simulink library "xpclib"  (Simulink 6.0)
settings: Solver=ode45  SolverMode=SingleTasking  StartTime=0.0  StopTime=10.0  RelTol=1e-3
values from neighbouring files (symbols this model uses):
  base = get_param( gcb, 'base' )    [maddiamondmm.m]    (also in maddiamondmm32frame.m; maddsmm16at.m; mdadsmm16at.m; mdiortddm64x0.m = hex2dec(addr(3:end)))
  block = find_system(bdroot,                          'FollowLinks', 'on',                          'LookUnderMasks', 'all',                          'MaskType', type )    [mdionipci6527.m]
  count = count + 1    (= 5)    [mdecodestate.m]
  port = get_param( gcb, 'port' )    [mdionipci6527.m]    (also in mdiortddm64x0.m = get_param(blocks{i}, 'port'))
undefined symbols (not defined in the file or in its folder): CIO, devid, DIO24, genixlib, get, handlers, irq, mbaseserialmask, mbwaudpmc, mdacbpcidas, mdiamondemeraldmask, mgenix, mmodemcontrol, mquamask, mrs232, msc150checks, mtargetboxleds, mtargetboxwatchdog, mxpccan, PCI, sizeof, vendid
libraries: xpclib x384, simulink x6
(part 6 of 7)

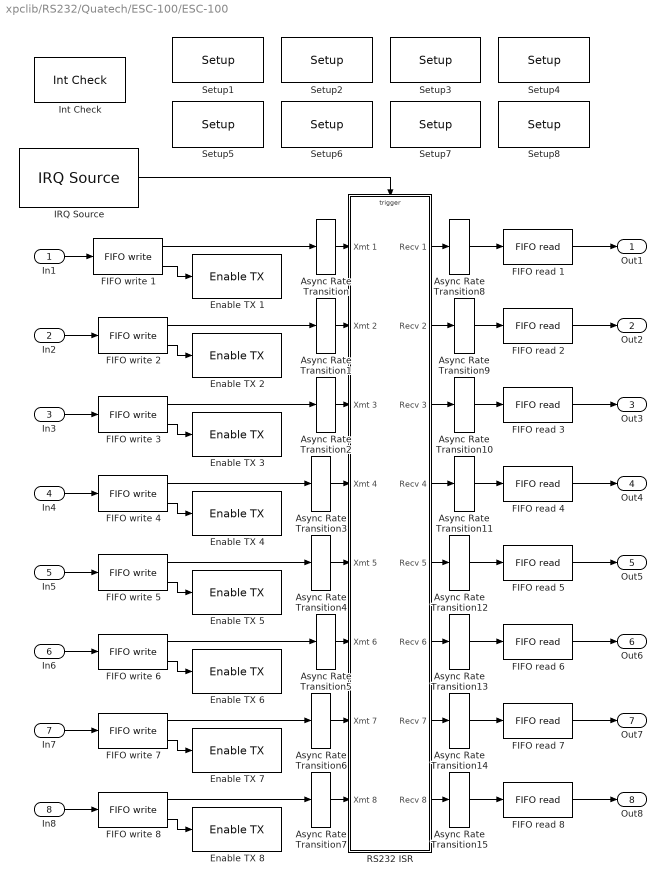
== system xpclib/RS232/Quatech/ESC-100/ESC-100 ==
  In1 : Inport  LatchInput=off
  In2 : Inport  Port=2  LatchInput=off
  In3 : Inport  Port=3  LatchInput=off
  In4 : Inport  Port=4  LatchInput=off
  In5 : Inport  Port=5  LatchInput=off
  In6 : Inport  Port=6  LatchInput=off
  In7 : Inport  Port=7  LatchInput=off
  In8 : Inport  Port=8  LatchInput=off
  Async Rate Transition{,1..15} (16 alike) : xpclib/Asynchronous Event/Async Rate Transition  sample_time=-1
  Enable TX 1 : xpclib/RS232/Quatech/ESC-100/ESC-100 Internal blocks/Enable TX   port=1  slot=brdslot
  Enable TX 2 : xpclib/RS232/Quatech/ESC-100/ESC-100 Internal blocks/Enable TX   port=2  slot=brdslot
  Enable TX 3 : xpclib/RS232/Quatech/ESC-100/ESC-100 Internal blocks/Enable TX   port=3  slot=brdslot
  Enable TX 4 : xpclib/RS232/Quatech/ESC-100/ESC-100 Internal blocks/Enable TX   port=4  slot=brdslot
  Enable TX 5 : xpclib/RS232/Quatech/ESC-100/ESC-100 Internal blocks/Enable TX   port=5  slot=brdslot
  Enable TX 6 : xpclib/RS232/Quatech/ESC-100/ESC-100 Internal blocks/Enable TX   port=6  slot=brdslot
  Enable TX 7 : xpclib/RS232/Quatech/ESC-100/ESC-100 Internal blocks/Enable TX   port=7  slot=brdslot
  Enable TX 8 : xpclib/RS232/Quatech/ESC-100/ESC-100 Internal blocks/Enable TX   port=8  slot=brdslot
  FIFO read {1..8} (8 alike) : xpclib/RS232/FIFO read   maxsize=1024  minsize=1  usedelimiter=on  delimiter=13  outputtype=count+16 bit uint  enable=off  enableout=off  sampletime=-1
  FIFO write 1 : xpclib/RS232/FIFO write   size=1024  inputtype=8 bit uint null terminated  present=on  sampletime=-1  id=XMT channel 1, IRQ 7
  FIFO write 2 : xpclib/RS232/FIFO write   size=1024  inputtype=8 bit uint null terminated  present=on  sampletime=-1  id=XMT channel 2, IRQ 7
  FIFO write 3 : xpclib/RS232/FIFO write   size=1024  inputtype=8 bit uint null terminated  present=on  sampletime=-1  id=XMT channel 3, IRQ 7
  FIFO write 4 : xpclib/RS232/FIFO write   size=1024  inputtype=8 bit uint null terminated  present=on  sampletime=-1  id=XMT channel 4, IRQ 7
  FIFO write 5 : xpclib/RS232/FIFO write   size=1024  inputtype=8 bit uint null terminated  present=on  sampletime=-1  id=XMT channel 5, IRQ 7
  FIFO write 6 : xpclib/RS232/FIFO write   size=1024  inputtype=8 bit uint null terminated  present=on  sampletime=-1  id=XMT channel 6, IRQ 7
  FIFO write 7 : xpclib/RS232/FIFO write   size=1024  inputtype=8 bit uint null terminated  present=on  sampletime=-1  id=XMT channel 7, IRQ 7
  FIFO write 8 : xpclib/RS232/FIFO write   size=1024  inputtype=8 bit uint null terminated  present=on  sampletime=-1  id=XMT channel 8, IRQ 7
  IRQ Source : xpclib/Asynchronous Event/IRQ Source  irqNo=7  preempt=off  b_type=None/Other  slot=brdslot
  Int Check : xpclib/RS232/Quatech/ESC-100/ESC-100 Internal blocks/Int Check  slot=brdslot  irqnum=7
  RS232 ISR : Subsystem  TreatAsAtomicUnit=on  PropExecContextAcrossSSBoundary=on  mask(RS232 ISR){slot=brdslot}
      mask help:
      | ESC-100
      | Quatech
      | Interrupt Service Routine
      mask init:
      | subslot = slot;
      mask Display:
      | disp('ESC-100\nISR');
      | port_label('input', 1, 'XMT1');
      | port_label('input', 2, 'XMT2');
      | port_label('input', 3, 'XMT3');
      | port_label('input', 4, 'XMT4');
      | port_label('input', 5, 'XMT5');
      | port_label('input', 6, 'XMT6');
      | port_label('input', 7, 'XMT7');
      | port_label('input', 8, 'XMT8');
      | port_label('output', 1, 'RCV1');
      | port_label('output', 2, 'RCV2');
      | port_label('output', 3, 'RCV3');
      | port_label('output', 4, 'RCV4');
      | port_label('output', 5, 'RCV5');
      | port_label('output', 6, 'RCV6');
      | port_label('output', 7, 'RCV7');
      | port_label('output', 8, 'RCV8');
  Setup1 : xpclib/RS232/Quatech/ESC-100/ESC-100 Internal blocks/Setup  port=1  baud=19200  width=8  nstop=1  parity=None  fmode=64 deep  rlevel=half full  ctsmode=on  slot=brdslot
  Setup2 : xpclib/RS232/Quatech/ESC-100/ESC-100 Internal blocks/Setup  port=2  baud=19200  width=8  nstop=1  parity=None  fmode=64 deep  rlevel=half full  ctsmode=on  slot=brdslot
  Setup3 : xpclib/RS232/Quatech/ESC-100/ESC-100 Internal blocks/Setup  port=3  baud=19200  width=8  nstop=1  parity=None  fmode=64 deep  rlevel=half full  ctsmode=on  slot=brdslot
  Setup4 : xpclib/RS232/Quatech/ESC-100/ESC-100 Internal blocks/Setup  port=4  baud=19200  width=8  nstop=1  parity=None  fmode=64 deep  rlevel=half full  ctsmode=on  slot=brdslot
  Setup5 : xpclib/RS232/Quatech/ESC-100/ESC-100 Internal blocks/Setup  port=5  baud=19200  width=8  nstop=1  parity=None  fmode=64 deep  rlevel=half full  ctsmode=on  slot=brdslot
  Setup6 : xpclib/RS232/Quatech/ESC-100/ESC-100 Internal blocks/Setup  port=6  baud=19200  width=8  nstop=1  parity=None  fmode=64 deep  rlevel=half full  ctsmode=on  slot=brdslot
  Setup7 : xpclib/RS232/Quatech/ESC-100/ESC-100 Internal blocks/Setup  port=7  baud=19200  width=8  nstop=1  parity=None  fmode=64 deep  rlevel=half full  ctsmode=on  slot=brdslot
  Setup8 : xpclib/RS232/Quatech/ESC-100/ESC-100 Internal blocks/Setup  port=8  baud=19200  width=8  nstop=1  parity=None  fmode=64 deep  rlevel=half full  ctsmode=on  slot=brdslot
  Out1 : Outport
  Out2 : Outport  Port=2
  Out3 : Outport  Port=3
  Out4 : Outport  Port=4
  Out5 : Outport  Port=5
  Out6 : Outport  Port=6
  Out7 : Outport  Port=7
  Out8 : Outport  Port=8
  wires:
  RS232 ISR/8(Recv 8) -> Async Rate Transition15/1
  RS232 ISR/7(Recv 7) -> Async Rate Transition14/1
  RS232 ISR/6(Recv 6) -> Async Rate Transition13/1
  RS232 ISR/5(Recv 5) -> Async Rate Transition12/1
  Async Rate Transition15/1 -> FIFO read 8/1
  FIFO read 8/1 -> Out8/1
  Async Rate Transition14/1 -> FIFO read 7/1
  FIFO read 7/1 -> Out7/1
  Async Rate Transition13/1 -> FIFO read 6/1
  FIFO read 6/1 -> Out6/1
  Async Rate Transition12/1 -> FIFO read 5/1
  FIFO read 5/1 -> Out5/1
  Async Rate Transition4/1 -> RS232 ISR/5(Xmt 5)
  Async Rate Transition5/1 -> RS232 ISR/6(Xmt 6)
  Async Rate Transition6/1 -> RS232 ISR/7(Xmt 7)
  Async Rate Transition7/1 -> RS232 ISR/8(Xmt 8)
  RS232 ISR/4(Recv 4) -> Async Rate Transition11/1
  Async Rate Transition1/1 -> RS232 ISR/2(Xmt 2)
  Async Rate Transition11/1 -> FIFO read 4/1
  Async Rate Transition10/1 -> FIFO read 3/1
  FIFO read 4/1 -> Out4/1
  FIFO read 3/1 -> Out3/1
  FIFO read 2/1 -> Out2/1
  Async Rate Transition9/1 -> FIFO read 2/1
  FIFO read 1/1 -> Out1/1
  Async Rate Transition8/1 -> FIFO read 1/1
  RS232 ISR/3(Recv 3) -> Async Rate Transition10/1
  RS232 ISR/2(Recv 2) -> Async Rate Transition9/1
  RS232 ISR/1(Recv 1) -> Async Rate Transition8/1
  Async Rate Transition3/1 -> RS232 ISR/4(Xmt 4)
  Async Rate Transition2/1 -> RS232 ISR/3(Xmt 3)
  Async Rate Transition/1 -> RS232 ISR/1(Xmt 1)
  IRQ Source/1 -> RS232 ISR/Trigger
  In1/1 -> FIFO write 1/1
  FIFO write 1/1 -> Async Rate Transition/1
  FIFO write 1/2 -> Enable TX 1/1
  FIFO write 2/1 -> Async Rate Transition1/1
  FIFO write 3/1 -> Async Rate Transition2/1
  FIFO write 4/1 -> Async Rate Transition3/1
  FIFO write 5/1 -> Async Rate Transition4/1
  FIFO write 6/1 -> Async Rate Transition5/1
  FIFO write 7/1 -> Async Rate Transition6/1
  FIFO write 8/1 -> Async Rate Transition7/1
  FIFO write 2/2 -> Enable TX 2/1
  FIFO write 3/2 -> Enable TX 3/1
  FIFO write 4/2 -> Enable TX 4/1
  FIFO write 5/2 -> Enable TX 5/1
  FIFO write 6/2 -> Enable TX 6/1
  FIFO write 7/2 -> Enable TX 7/1
  FIFO write 8/2 -> Enable TX 8/1
  In2/1 -> FIFO write 2/1
  In3/1 -> FIFO write 3/1
  In4/1 -> FIFO write 4/1
  In5/1 -> FIFO write 5/1
  In6/1 -> FIFO write 6/1
  In7/1 -> FIFO write 7/1
  In8/1 -> FIFO write 8/1

== system xpclib/RS232/Quatech/ESC-100/ESC-100 Internal blocks ==
  "Enable TX " : S-Function  FunctionName=sertxenable  Parameters=slot, port, 2  mask(Enable TX Int){port=1, slot=-1}
      mask prompts: slot "PCI slot: (-1 for autosearch)"
      mask help:
      | ESC-100
      | Quatech
      | Enable TX Interrupt
      mask Help: helpview(fullfile(docroot, 'mapfiles', 'xpc.map'), 'Quatech_Enable_Int')
      mask StyleString: popup(1|2|3|4|5|6|7|8),edit
      mask Display:
      | disp('ESC-100\nQuatech\nEnable TX int');
      | port_label('input', 1, 'E');
  Filter Int Reason : S-Function  FunctionName=filterqua  Parameters=port, 2, value  mask(Interrupt Source Filter){port=1, value=Transmitter empty}
      mask prompts: value "Filter value:"
      mask help:
      | ESC-100
      | Quatech
      | Interrupt Source Filter
      mask Help: helpview(fullfile(docroot, 'mapfiles', 'xpc.map'), 'Quatech_Filter_Ints')
      mask StyleString: popup(1|2|3|4|5|6|7|8),popup(Receive data|Transmitter empty|Modem status change)
      mask Display:
      | disp('ESC-100\nQuatech\nFilter Int Reason');
      | port_label('input', 1, 'S' );
      | port_label('output', 1, 'E' );
  Int Check : S-Function  FunctionName=intcheckqua  Parameters=slot, irqnum+4, boardtype,  mask(interrupt check){slot=-1, irqnum=5}
      mask prompts: slot "PCI slot: (-1 for autosearch)"; irqnum "IRQ Line Number"
      mask help:
      | ESC-100
      | Quatech
      | Interrupt Check
      mask init:
      | boardtype = 2;
      mask Help: helpview(fullfile(docroot, 'mapfiles', 'xpc.map'), 'Quatech_Interrupt_Check')
      mask StyleString: edit,popup(5|6|7|8|9|10|11|12|13|14|15)
      mask Display: disp('ESC-100\nQuatech\nInterrupt Check');
  Read HW FIFO : S-Function  FunctionName=serreadqua  Parameters=slot, port, 2, flush  mask(Read Data Port){port=1, flush=on, slot=-1}
      mask prompts: flush "Flush HW FIFO on startup"; slot "PCI slot: (-1 for autosearch)"
      mask help:
      | ESC-100
      | Quatech
      | Read Data Port
      mask Help: helpview(fullfile(docroot, 'mapfiles', 'xpc.map'), 'Quatech_Read_HW')
      mask StyleString: popup(1|2|3|4|5|6|7|8),checkbox,edit
      mask Display:
      | disp('ESC-100\nQuatech\nRead HW FIFO');
      | port_label('input', 1, 'E');
      | port_label('output', 1, 'D');
  Read Int Status : S-Function  FunctionName=iqueryqua  Parameters=slot, 2  mask(Interrupt Query){slot=-1}
      mask prompts: slot "PCI slot: (-1 for autosearch)"
      mask help:
      | ESC-100
      | Quatech
      | Interrupt Query
      mask Help: helpview(fullfile(docroot, 'mapfiles', 'xpc.map'), 'Quatech_Interrupt_Query')
      mask Display:
      | disp('ESC-100\nQuatech\nRead Int Status');
      | port_label('output', 1, 'S' );
  Setup : S-Function  FunctionName=setupqua  Parameters=slot, boardtype, port, baud, width, nstop, parity, fmode, ctsmode, rlevel  mask(setup){port=1, baud=115200, width=8, nstop=1, parity=None, fmode=64 deep, rlevel=half full, ctsmode=off, slot=-1}
      mask prompts: baud "Baud rate:"; width "Number of data bits:"; nstop "Number of stop bits:"; fmode "Fifo mode:"; rlevel "Receive trigger level:"; ctsmode "Enable auto RTS/CTS"; slot "PCI slot: (-1 for autosearch)"
      mask help:
      | ESC-100
      | Quatech
      | Setup
      mask init:
      | boardtype = 2;
      mask Help: helpview(fullfile(docroot, 'mapfiles', 'xpc.map'), 'Quatech_Setup')
      mask StyleString: popup(1|2|3|4|5|6|7|8),popup(921600|460800|230400|115200|57600|38400|19200|9600|4800|2400|1200|600|300|110),popup(5|6|7|8),popup(1|2),popup(None|Even|Odd|Mark|Space),popup(64 deep|16 deep|1 deep),popup(1|quarter full|half full|almost full),checkbox,edit
      mask Display: disp('ESC-100\nQuatech\nSetup')
  Write HW FIFO : S-Function  FunctionName=serwritequa  Parameters=slot, port, 2, 0  mask(Write Data Port){port=1, slot=-1}
      mask prompts: slot "PCI slot: (-1 for autosearch)"
      mask help:
      | ESC-100
      | Quatech
      | Write Data Port
      mask Help: helpview(fullfile(docroot, 'mapfiles', 'xpc.map'), 'Quatech_Write_HW')
      mask StyleString: popup(1|2|3|4|5|6|7|8),edit
      mask Display:
      | disp('ESC-100\nQuatech\nWrite HW FIFO');
      | port_label('input', 1, 'D');
      | port_label('input', 2, 'E');

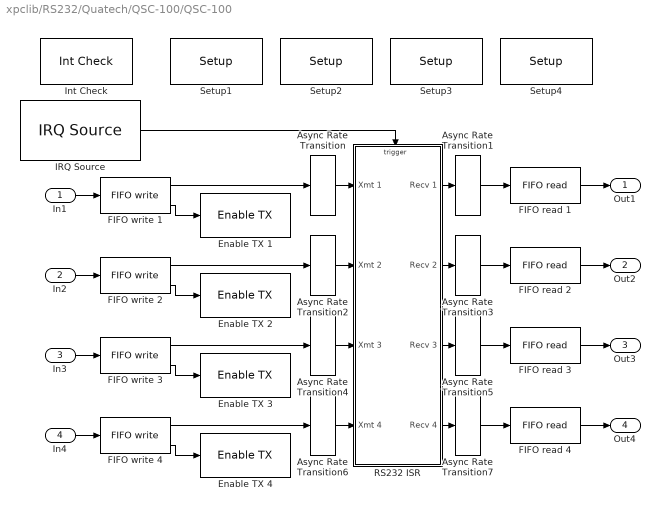
== system xpclib/RS232/Quatech/QSC-100/QSC-100 ==
  In1 : Inport  LatchInput=off
  In2 : Inport  Port=2  LatchInput=off
  In3 : Inport  Port=3  LatchInput=off
  In4 : Inport  Port=4  LatchInput=off
  Async Rate Transition{,1..7} (8 alike) : xpclib/Asynchronous Event/Async Rate Transition  sample_time=-1
  Enable TX 1 : xpclib/RS232/Quatech/QSC-100/QSC-100 Internal  blocks/Enable TX   port=1  slot=brdslot
  Enable TX 2 : xpclib/RS232/Quatech/QSC-100/QSC-100 Internal  blocks/Enable TX   port=2  slot=brdslot
  Enable TX 3 : xpclib/RS232/Quatech/QSC-100/QSC-100 Internal  blocks/Enable TX   port=3  slot=brdslot
  Enable TX 4 : xpclib/RS232/Quatech/QSC-100/QSC-100 Internal  blocks/Enable TX   port=4  slot=brdslot
  FIFO read {1..4} (4 alike) : xpclib/RS232/FIFO read   maxsize=1024  minsize=1  usedelimiter=on  delimiter=13  outputtype=count+16 bit uint  enable=off  enableout=off  sampletime=-1
  FIFO write 1 : xpclib/RS232/FIFO write   size=1024  inputtype=8 bit uint null terminated  present=on  sampletime=-1  id=XMT channel 1, IRQ 7
  FIFO write 2 : xpclib/RS232/FIFO write   size=1024  inputtype=8 bit uint null terminated  present=on  sampletime=-1  id=XMT channel 2, IRQ 7
  FIFO write 3 : xpclib/RS232/FIFO write   size=1024  inputtype=8 bit uint null terminated  present=on  sampletime=-1  id=XMT channel 3, IRQ 7
  FIFO write 4 : xpclib/RS232/FIFO write   size=1024  inputtype=8 bit uint null terminated  present=on  sampletime=-1  id=XMT channel 4, IRQ 7
  IRQ Source : xpclib/Asynchronous Event/IRQ Source  irqNo=7  preempt=off  b_type=None/Other  slot=brdslot
  Int Check : xpclib/RS232/Quatech/QSC-100/QSC-100 Internal  blocks/Int Check  slot=brdslot  irqnum=7
  RS232 ISR : Subsystem  TreatAsAtomicUnit=on  PropExecContextAcrossSSBoundary=on  mask(RS232 ISR){slot=brdslot}
      mask help:
      | QSC-100
      | Quatech
      | Interrupt Service Routine
      mask init:
      | subslot = slot;
      mask Display:
      | disp('QSC-100\nISR');
      | port_label('input', 1, 'XMT1');
      | port_label('input', 2, 'XMT2');
      | port_label('input', 3, 'XMT3');
      | port_label('input', 4, 'XMT4');
      | port_label('output', 1, 'RCV1');
      | port_label('output', 2, 'RCV2');
      | port_label('output', 3, 'RCV3');
      | port_label('output', 4, 'RCV4');
  Setup1 : xpclib/RS232/Quatech/QSC-100/QSC-100 Internal  blocks/Setup  port=1  baud=115200  width=8  nstop=1  parity=None  fmode=64 deep  rlevel=half full  ctsmode=on  slot=brdslot
  Setup2 : xpclib/RS232/Quatech/QSC-100/QSC-100 Internal  blocks/Setup  port=2  baud=115200  width=8  nstop=1  parity=None  fmode=64 deep  rlevel=half full  ctsmode=on  slot=brdslot
  Setup3 : xpclib/RS232/Quatech/QSC-100/QSC-100 Internal  blocks/Setup  port=3  baud=115200  width=8  nstop=1  parity=None  fmode=64 deep  rlevel=half full  ctsmode=on  slot=brdslot
  Setup4 : xpclib/RS232/Quatech/QSC-100/QSC-100 Internal  blocks/Setup  port=4  baud=115200  width=8  nstop=1  parity=None  fmode=64 deep  rlevel=half full  ctsmode=on  slot=brdslot
  Out1 : Outport
  Out2 : Outport  Port=2
  Out3 : Outport  Port=3
  Out4 : Outport  Port=4
  wires:
  FIFO write 1/2 -> Enable TX 1/1
  IRQ Source/1 -> RS232 ISR/Trigger
  Async Rate Transition/1 -> RS232 ISR/1(Xmt 1)
  Async Rate Transition4/1 -> RS232 ISR/3(Xmt 3)
  Async Rate Transition6/1 -> RS232 ISR/4(Xmt 4)
  RS232 ISR/1(Recv 1) -> Async Rate Transition1/1
  RS232 ISR/2(Recv 2) -> Async Rate Transition3/1
  RS232 ISR/3(Recv 3) -> Async Rate Transition5/1
  FIFO write 1/1 -> Async Rate Transition/1
  In1/1 -> FIFO write 1/1
  FIFO write 2/1 -> Async Rate Transition2/1
  FIFO write 3/1 -> Async Rate Transition4/1
  FIFO write 4/1 -> Async Rate Transition6/1
  In4/1 -> FIFO write 4/1
  In3/1 -> FIFO write 3/1
  In2/1 -> FIFO write 2/1
  Async Rate Transition1/1 -> FIFO read 1/1
  FIFO read 1/1 -> Out1/1
  Async Rate Transition3/1 -> FIFO read 2/1
  FIFO read 2/1 -> Out2/1
  FIFO read 3/1 -> Out3/1
  FIFO read 4/1 -> Out4/1
  Async Rate Transition5/1 -> FIFO read 3/1
  Async Rate Transition7/1 -> FIFO read 4/1
  FIFO write 2/2 -> Enable TX 2/1
  FIFO write 3/2 -> Enable TX 3/1
  FIFO write 4/2 -> Enable TX 4/1
  Async Rate Transition2/1 -> RS232 ISR/2(Xmt 2)
  RS232 ISR/4(Recv 4) -> Async Rate Transition7/1

== system xpclib/RS232/Quatech/QSC-100/QSC-100 Internal  blocks ==
  "Enable TX " : S-Function  FunctionName=sertxenable  Parameters=slot, port, 1  mask(Enable TX Int){port=1, slot=-1}
      mask prompts: slot "PCI slot: (-1 for autosearch)"
      mask help:
      | QSC-100
      | Quatech
      | Enable TX Interrupt
      mask Help: helpview(fullfile(docroot, 'mapfiles', 'xpc.map'), 'Quatech_Enable_Int')
      mask StyleString: popup(1|2|3|4),edit
      mask Display:
      | disp('QSC-100\nQuatech\nEnable TX int');
      | port_label('input', 1, 'E');
  Filter Int Reason : S-Function  FunctionName=filterqua  Parameters=port, 1, value  mask(Interrupt Source Filter){port=1, value=Receive data}
      mask prompts: value "Filter value:"
      mask help:
      | QSC-100
      | Quatech
      | Interrupt Source Filter
      mask Help: helpview(fullfile(docroot, 'mapfiles', 'xpc.map'), 'Quatech_Filter_Ints')
      mask StyleString: popup(1|2|3|4),popup(Receive data|Transmitter empty|Modem status change)
      mask Display:
      | disp('QSC-100\nQuatech\nFilter Int Reason');
      | port_label('input', 1, 'S' );
      | port_label('output', 1, 'E' );
  Int Check : S-Function  FunctionName=intcheckqua  Parameters=slot, irqnum+4, boardtype,  mask(interrupt check){slot=-1, irqnum=5}
      mask prompts: slot "PCI slot: (-1 for autosearch)"; irqnum "IRQ Line Number"
      mask help:
      | QSC-100
      | Quatech
      | Interrupt Check
      mask init:
      | boardtype = 1;
      mask Help: helpview(fullfile(docroot, 'mapfiles', 'xpc.map'), 'Quatech_Interrupt_Check')
      mask StyleString: edit,popup(5|6|7|8|9|10|11|12|13|14|15)
      mask Display: disp('QSC-100\nQuatech\nInterrupt Check');
  Read HW FIFO : S-Function  FunctionName=serreadqua  Parameters=slot, port, 1, flush  mask(Read Data Port){port=1, flush=on, slot=-1}
      mask prompts: flush "Flush HW FIFO on startup"; slot "PCI slot: (-1 for autosearch)"
      mask help:
      | QSC-100
      | Quatech
      | Read Data Port
      mask Help: helpview(fullfile(docroot, 'mapfiles', 'xpc.map'), 'Quatech_Read_HW')
      mask StyleString: popup(1|2|3|4),checkbox,edit
      mask Display:
      | disp('QSC-100\nQuatech\nRead HW FIFO');
      | port_label('input', 1, 'E');
      | port_label('output', 1, 'D');
  Read Int Status : S-Function  FunctionName=iqueryqua  Parameters=slot, 1  mask(Interrupt Query){slot=-1}
      mask prompts: slot "PCI slot: (-1 for autosearch)"
      mask help:
      | QSC-100
      | Quatech
      | Interrupt Query
      mask Help: helpview(fullfile(docroot, 'mapfiles', 'xpc.map'), 'Quatech_Interrupt_Query')
      mask Display:
      | disp('QSC-100\nQuatech\nRead Int Status');
      | port_label('output', 1, 'S' );
  Setup : S-Function  FunctionName=setupqua  Parameters=slot, boardtype, port, baud, width, nstop, parity, fmode, ctsmode, rlevel  mask(setup){port=1, baud=115200, width=8, nstop=1, parity=None, fmode=64 deep, rlevel=half full, ctsmode=off, slot=-1}
      mask prompts: baud "Baud rate:"; width "Number of data bits:"; nstop "Number of stop bits:"; fmode "Fifo mode:"; rlevel "Receive trigger level:"; ctsmode "Enable auto RTS/CTS"; slot "PCI slot: (-1 for autosearch)"
      mask help:
      | QSC-100
      | Quatech
      | Setup
      mask init:
      | boardtype = 1;
      mask Help: helpview(fullfile(docroot, 'mapfiles', 'xpc.map'), 'Quatech_Setup')
      mask StyleString: popup(1|2|3|4),popup(921600|460800|230400|115200|57600|38400|19200|9600|4800|2400|1200|600|300|110),popup(5|6|7|8),popup(1|2),popup(None|Even|Odd|Mark|Space),popup(64 deep|16 deep|1 deep),popup(1|quarter full|half full|almost full),checkbox,edit
      mask Display: disp('QSC-100\nQuatech\nSetup');
  Write HW FIFO : S-Function  FunctionName=serwritequa  Parameters=slot, port, 1, 0  mask(Write Data Port){port=1, slot=-1}
      mask prompts: slot "PCI slot: (-1 for autosearch)"
      mask help:
      | QSC-100
      | Quatech
      | Write Data Port
      mask Help: helpview(fullfile(docroot, 'mapfiles', 'xpc.map'), 'Quatech_Write_HW')
      mask StyleString: popup(1|2|3|4),edit
      mask Display:
      | disp('QSC-100\nQuatech\nWrite HW FIFO');
      | port_label('input', 1, 'D');
      | port_label('input', 2, 'E');

== system xpclib/RS232/Quatech/QSC-200/300/QSC-200/300 Internal  blocks1 ==
  "Enable TX " : S-Function  FunctionName=sertxenable  Parameters=slot, port, 3  mask(Enable TX Int){port=1, slot=-1}
      mask prompts: slot "PCI slot: (-1 for autosearch)"
      mask help:
      | QSC-200/300
      | Quatech
      | Enable TX Interrupt
      mask Help: helpview(fullfile(docroot, 'mapfiles', 'xpc.map'), 'Quatech_Enable_Int')
      mask StyleString: popup(1|2|3|4),edit
      mask Display:
      | disp('QSC-200/300\nQuatech\nEnable TX int');
      | port_label('input', 1, 'E');
  Filter Int Reason : S-Function  FunctionName=filterqua  Parameters=port, 3, value  mask(Interrupt Source Filter){port=1, value=Receive data}
      mask prompts: value "Filter value:"
      mask help:
      | QSC-200/300
      | Quatech
      | Interrupt Source Filter
      mask Help: helpview(fullfile(docroot, 'mapfiles', 'xpc.map'), 'Quatech_Filter_Ints')
      mask StyleString: popup(1|2|3|4),popup(Receive data|Transmitter empty|Modem status change)
      mask Display:
      | disp('QSC-200/300\nQuatech\nFilter Int Reason');
      | port_label('input', 1, 'S' );
      | port_label('output', 1, 'E' );
  Int Check : S-Function  FunctionName=intcheckqua  Parameters=slot, irqnum+4, boardtype,  mask(interrupt check){slot=-1, irqnum=5}
      mask prompts: slot "PCI slot: (-1 for autosearch)"; irqnum "IRQ Line Number"
      mask help:
      | QSC-200/300
      | Quatech
      | Interrupt Check
      mask init:
      | boardtype = 3;
      mask Help: helpview(fullfile(docroot, 'mapfiles', 'xpc.map'), 'Quatech_Interrupt_Check')
      mask StyleString: edit,popup(5|6|7|8|9|10|11|12|13|14|15)
      mask Display: disp('QSC-200/300\nQuatech\nInterrupt Check');
  Read HW FIFO : S-Function  FunctionName=serreadqua  Parameters=slot, port, 3, flush  mask(Read Data Port){port=1, flush=on, slot=-1}
      mask prompts: flush "Flush HW FIFO on startup"; slot "PCI slot: (-1 for autosearch)"
      mask help:
      | QSC-200/300
      | Quatech
      | Read Data Port
      mask Help: helpview(fullfile(docroot, 'mapfiles', 'xpc.map'), 'Quatech_Read_HW')
      mask StyleString: popup(1|2|3|4),checkbox,edit
      mask Display:
      | disp('QSC-200/300\nQuatech\nRead HW FIFO');
      | port_label('input', 1, 'E');
      | port_label('output', 1, 'D');
  Read Int Status : S-Function  FunctionName=iqueryqua  Parameters=slot, 3  mask(Interrupt Query){slot=-1}
      mask prompts: slot "PCI slot: (-1 for autosearch)"
      mask help:
      | QSC-200/300
      | Quatech
      | Interrupt Query
      mask Help: helpview(fullfile(docroot, 'mapfiles', 'xpc.map'), 'Quatech_Interrupt_Query')
      mask Display:
      | disp('QSC-200/300\nQuatech\nRead Int Status');
      | port_label('output', 1, 'S' );
  Setup : S-Function  FunctionName=setupqua  Parameters=slot, boardtype, port, baud, width, nstop, parity, fmode, ctsmode, rlevel  mask(setup){port=1, baud=115200, width=8, nstop=1, parity=None, fmode=64 deep, rlevel=half full, ctsmode=off, slot=-1}
      mask prompts: baud "Baud rate:"; width "Number of data bits:"; nstop "Number of stop bits:"; fmode "Fifo mode:"; rlevel "Receive trigger level:"; ctsmode "Enable auto RTS/CTS"; slot "PCI slot: (-1 for autosearch)"
      mask help:
      | QSC-200/300
      | Quatech
      | Setup
      mask init:
      | boardtype = 3;
      mask Help: helpview(fullfile(docroot, 'mapfiles', 'xpc.map'), 'Quatech_Setup')
      mask StyleString: popup(1|2|3|4),popup(921600|460800|230400|115200|57600|38400|19200|9600|4800|2400|1200|600|300|110),popup(5|6|7|8),popup(1|2),popup(None|Even|Odd|Mark|Space),popup(64 deep|16 deep|1 deep),popup(1|quarter full|half full|almost full),checkbox,edit
      mask Display: disp('QSC-200/300\nQuatech\nSetup');
  Write HW FIFO : S-Function  FunctionName=serwritequa  Parameters=slot, port, 3, onxmt  mask(Write Data Port){port=1, onxmt=None, slot=-1}
      mask prompts: onxmt "Assert on Transmit:"; slot "PCI slot: (-1 for autosearch)"
      mask help:
      | QSC-200/300
      | Quatech
      | Write Data Port
      mask Help: helpview(fullfile(docroot, 'mapfiles', 'xpc.map'), 'Quatech_Write_HW')
      mask StyleString: popup(1|2|3|4),popup(None|RTS|DTR),edit
      mask Display:
      | disp('QSC-200/300\nQuatech\nWrite HW FIFO');
      | port_label('input', 1, 'D');
      | port_label('input', 2, 'E');

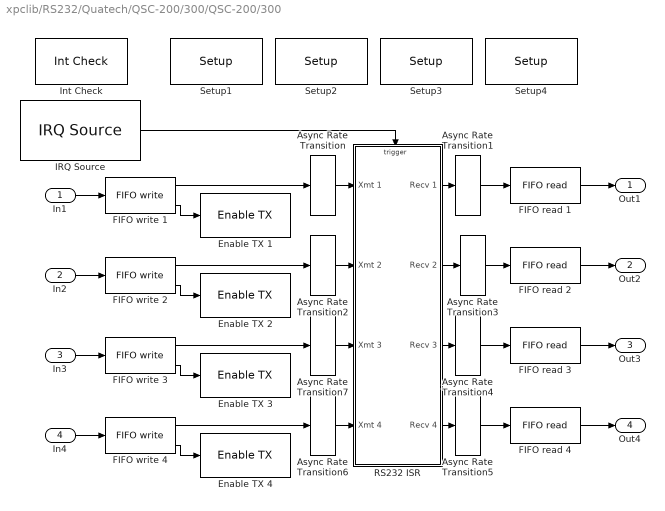
== system xpclib/RS232/Quatech/QSC-200/300/QSC-200/300  ==
  In1 : Inport  LatchInput=off
  In2 : Inport  Port=2  LatchInput=off
  In3 : Inport  Port=3  LatchInput=off
  In4 : Inport  Port=4  LatchInput=off
  Async Rate Transition{,1..7} (8 alike) : xpclib/Asynchronous Event/Async Rate Transition  sample_time=-1
  Enable TX 1 : xpclib/RS232/Quatech/QSC-200//300/QSC-200//300 Internal  blocks1/Enable TX   port=1  slot=brdslot
  Enable TX 2 : xpclib/RS232/Quatech/QSC-200//300/QSC-200//300 Internal  blocks1/Enable TX   port=2  slot=brdslot
  Enable TX 3 : xpclib/RS232/Quatech/QSC-200//300/QSC-200//300 Internal  blocks1/Enable TX   port=3  slot=brdslot
  Enable TX 4 : xpclib/RS232/Quatech/QSC-200//300/QSC-200//300 Internal  blocks1/Enable TX   port=4  slot=brdslot
  FIFO read {1..4} (4 alike) : xpclib/RS232/FIFO read   maxsize=1024  minsize=1  usedelimiter=on  delimiter=13  outputtype=count+16 bit uint  enable=off  enableout=off  sampletime=-1
  FIFO write {1..4} (4 alike) : xpclib/RS232/FIFO write   size=1024  inputtype=8 bit uint null terminated  present=on  sampletime=-1
  IRQ Source : xpclib/Asynchronous Event/IRQ Source  irqNo=7  preempt=off  b_type=None/Other  slot=brdslot
  Int Check : xpclib/RS232/Quatech/QSC-200//300/QSC-200//300 Internal  blocks1/Int Check  slot=brdslot  irqnum=7
  RS232 ISR : Subsystem  TreatAsAtomicUnit=on  PropExecContextAcrossSSBoundary=on  mask(RS232 ISR){slot=brdslot}
      mask help:
      | QSC-100
      | Quatech
      | Interrupt Service Routine
      mask init:
      | subslot = slot;
      mask Display:
      | disp('QSC-100\nISR');
      | port_label('input', 1, 'XMT1');
      | port_label('input', 2, 'XMT2');
      | port_label('input', 3, 'XMT3');
      | port_label('input', 4, 'XMT4');
      | port_label('output', 1, 'RCV1');
      | port_label('output', 2, 'RCV2');
      | port_label('output', 3, 'RCV3');
      | port_label('output', 4, 'RCV4');
  Setup1 : xpclib/RS232/Quatech/QSC-200//300/QSC-200//300 Internal  blocks1/Setup  port=1  baud=115200  width=8  nstop=1  parity=None  fmode=64 deep  rlevel=half full  ctsmode=on  slot=brdslot
  Setup2 : xpclib/RS232/Quatech/QSC-200//300/QSC-200//300 Internal  blocks1/Setup  port=2  baud=115200  width=8  nstop=1  parity=None  fmode=64 deep  rlevel=half full  ctsmode=on  slot=brdslot
  Setup3 : xpclib/RS232/Quatech/QSC-200//300/QSC-200//300 Internal  blocks1/Setup  port=3  baud=115200  width=8  nstop=1  parity=None  fmode=64 deep  rlevel=half full  ctsmode=on  slot=brdslot
  Setup4 : xpclib/RS232/Quatech/QSC-200//300/QSC-200//300 Internal  blocks1/Setup  port=4  baud=115200  width=8  nstop=1  parity=None  fmode=64 deep  rlevel=half full  ctsmode=on  slot=brdslot
  Out1 : Outport
  Out2 : Outport  Port=2
  Out3 : Outport  Port=3
  Out4 : Outport  Port=4
  wires:
  RS232 ISR/4(Recv 4) -> Async Rate Transition5/1
  Async Rate Transition2/1 -> RS232 ISR/2(Xmt 2)
  FIFO write 4/2 -> Enable TX 4/1
  FIFO write 3/2 -> Enable TX 3/1
  FIFO write 2/2 -> Enable TX 2/1
  FIFO read 4/1 -> Out4/1
  FIFO read 3/1 -> Out3/1
  FIFO read 2/1 -> Out2/1
  FIFO read 1/1 -> Out1/1
  Async Rate Transition1/1 -> FIFO read 1/1
  In2/1 -> FIFO write 2/1
  In3/1 -> FIFO write 3/1
  In4/1 -> FIFO write 4/1
  FIFO write 4/1 -> Async Rate Transition6/1
  FIFO write 3/1 -> Async Rate Transition7/1
  FIFO write 2/1 -> Async Rate Transition2/1
  In1/1 -> FIFO write 1/1
  FIFO write 1/1 -> Async Rate Transition/1
  RS232 ISR/3(Recv 3) -> Async Rate Transition4/1
  RS232 ISR/2(Recv 2) -> Async Rate Transition3/1
  RS232 ISR/1(Recv 1) -> Async Rate Transition1/1
  Async Rate Transition6/1 -> RS232 ISR/4(Xmt 4)
  Async Rate Transition7/1 -> RS232 ISR/3(Xmt 3)
  Async Rate Transition/1 -> RS232 ISR/1(Xmt 1)
  IRQ Source/1 -> RS232 ISR/Trigger
  FIFO write 1/2 -> Enable TX 1/1
  Async Rate Transition4/1 -> FIFO read 3/1
  Async Rate Transition5/1 -> FIFO read 4/1
  Async Rate Transition3/1 -> FIFO read 2/1

== system xpclib/RS232/Diamond/Emerald-MM /Diamond Emerald-MM Serial/RS232 ISR ==
  Xmt 1 : Inport  LatchInput=off
  Xmt 2 : Inport  Port=2  LatchInput=off
  Xmt 3 : Inport  Port=3  LatchInput=off
  Xmt 4 : Inport  Port=4  LatchInput=off
  function : TriggerPort  TriggerType=function-call
  While Iterator Subsystem : Subsystem  TreatAsAtomicUnit=on  PropExecContextAcrossSSBoundary=on
  Recv 1 : Outport
  Recv 2 : Outport  Port=2
  Recv 3 : Outport  Port=3
  Recv 4 : Outport  Port=4
  wires:
  While Iterator Subsystem/4(Recv 4) -> Recv 4/1
  While Iterator Subsystem/3(Recv 3) -> Recv 3/1
  Xmt 4/1 -> While Iterator Subsystem/4(Xmt 4)
  Xmt 3/1 -> While Iterator Subsystem/3(Xmt 3)
  While Iterator Subsystem/2(Recv 2) -> Recv 2/1
  While Iterator Subsystem/1(Recv 1) -> Recv 1/1
  Xmt 2/1 -> While Iterator Subsystem/2(Xmt 2)
  Xmt 1/1 -> While Iterator Subsystem/1(Xmt 1)

== system xpclib/RS232/Diamond/Emerald-MM8 /Diamond Emerald-MM8 Serial/RS232 ISR ==
  Xmt 1 : Inport  LatchInput=off
  Xmt 2 : Inport  Port=2  LatchInput=off
  Xmt 3 : Inport  Port=3  LatchInput=off
  Xmt 4 : Inport  Port=4  LatchInput=off
  Xmt 5 : Inport  Port=5  LatchInput=off
  Xmt 6 : Inport  Port=6  LatchInput=off
  Xmt 7 : Inport  Port=7  LatchInput=off
  Xmt 8 : Inport  Port=8  LatchInput=off
  function : TriggerPort  TriggerType=function-call
  While Iterator Subsystem : Subsystem  TreatAsAtomicUnit=on  PropExecContextAcrossSSBoundary=on
  Recv 1 : Outport
  Recv 2 : Outport  Port=2
  Recv 3 : Outport  Port=3
  Recv 4 : Outport  Port=4
  Recv 5 : Outport  Port=5
  Recv 6 : Outport  Port=6
  Recv 7 : Outport  Port=7
  Recv 8 : Outport  Port=8
  wires:
  Xmt 8/1 -> While Iterator Subsystem/8(Xmt 8)
  Xmt 7/1 -> While Iterator Subsystem/7(Xmt 7)
  Xmt 6/1 -> While Iterator Subsystem/6(Xmt 6)
  Xmt 5/1 -> While Iterator Subsystem/5(Xmt 5)
  While Iterator Subsystem/8(Recv 8) -> Recv 8/1
  While Iterator Subsystem/7(Recv 7) -> Recv 7/1
  While Iterator Subsystem/6(Recv 6) -> Recv 6/1
  While Iterator Subsystem/5(Recv 5) -> Recv 5/1
  While Iterator Subsystem/4(Recv 4) -> Recv 4/1
  While Iterator Subsystem/3(Recv 3) -> Recv 3/1
  Xmt 4/1 -> While Iterator Subsystem/4(Xmt 4)
  Xmt 3/1 -> While Iterator Subsystem/3(Xmt 3)
  While Iterator Subsystem/2(Recv 2) -> Recv 2/1
  While Iterator Subsystem/1(Recv 1) -> Recv 1/1
  Xmt 2/1 -> While Iterator Subsystem/2(Xmt 2)
  Xmt 1/1 -> While Iterator Subsystem/1(Xmt 1)

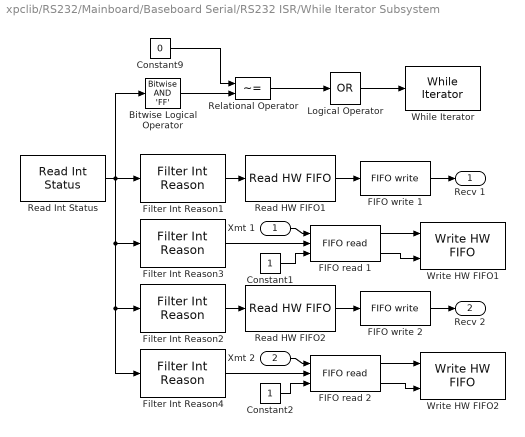
== system xpclib/RS232/Mainboard/Baseboard Serial/RS232 ISR/While Iterator Subsystem ==
  Xmt 1 : Inport  LatchInput=off
  Xmt 2 : Inport  Port=2  LatchInput=off
  Bitwise Logical Operator : simulink/Logic and Bit Operations/Bitwise Operator  logicop=AND  UseBitMask=on  BitMask='FF'  BitMaskRealWorld=Stored Integer
  Constant1 : Constant  OutDataTypeMode=uint32
  Constant2 : Constant  OutDataTypeMode=uint32
  Constant9 : Constant  Value=0  OutDataTypeMode=uint32
  FIFO read 1 : xpclib/RS232/FIFO read   maxsize=60  minsize=1  usedelimiter=off  delimiter=13  outputtype=count+32 bit uint  enable=on  enableout=on  sampletime=-1
  FIFO read 2 : xpclib/RS232/FIFO read   maxsize=60  minsize=1  usedelimiter=off  delimiter=13  outputtype=count+32 bit uint  enable=on  enableout=on  sampletime=-1
  FIFO write 1 : xpclib/RS232/FIFO write   size=1024  inputtype=count+32 bit uint  present=off  sampletime=-1  id=RCV channel 1, IRQ 4
  FIFO write 2 : xpclib/RS232/FIFO write   size=1024  inputtype=count+32 bit uint  present=off  sampletime=-1  id=RCV channel 2, IRQ 4
  Filter Int Reason1 : xpclib/RS232/Mainboard/Baseboard Serial Internal  blocks/Filter Int Reason  port=1  value=Receive data
  Filter Int Reason2 : xpclib/RS232/Mainboard/Baseboard Serial Internal  blocks/Filter Int Reason  port=2  value=Receive data
  Filter Int Reason3 : xpclib/RS232/Mainboard/Baseboard Serial Internal  blocks/Filter Int Reason  port=1  value=Transmitter empty
  Filter Int Reason4 : xpclib/RS232/Mainboard/Baseboard Serial Internal  blocks/Filter Int Reason  port=2  value=Transmitter empty
  Logical Operator : Logic  Operator=OR  Inputs=1  AllPortsSameDT=off
  Read HW FIFO1 : xpclib/RS232/Mainboard/Baseboard Serial Internal  blocks/Read HW FIFO  flush=on  addr=baddr1
  Read HW FIFO2 : xpclib/RS232/Mainboard/Baseboard Serial Internal  blocks/Read HW FIFO  flush=on  addr=baddr2
  Read Int Status : xpclib/RS232/Mainboard/Baseboard Serial Internal  blocks/Read Int Status  addr1=baddr1  addr2=baddr2
  Relational Operator : RelationalOperator  Operator=~=
  While Iterator : WhileIterator  MaxIters=65  WhileBlockType=do-while
  Write HW FIFO1 : xpclib/RS232/Mainboard/Baseboard Serial Internal  blocks/Write HW FIFO  addr=baddr1
  Write HW FIFO2 : xpclib/RS232/Mainboard/Baseboard Serial Internal  blocks/Write HW FIFO  addr=baddr2
  Recv 1 : Outport
  Recv 2 : Outport  Port=2
  wires:
  Read Int Status/1 -> Filter Int Reason1/1, Filter Int Reason3/1, Filter Int Reason4/1, Filter Int Reason2/1, Bitwise Logical Operator/1
  Filter Int Reason1/1 -> Read HW FIFO1/1
  FIFO write 1/1 -> Recv 1/1
  Read HW FIFO1/1 -> FIFO write 1/1
  Filter Int Reason3/1 -> FIFO read 1/2
  Xmt 1/1 -> FIFO read 1/1
  Filter Int Reason2/1 -> Read HW FIFO2/1
  FIFO write 2/1 -> Recv 2/1
  Read HW FIFO2/1 -> FIFO write 2/1
  Filter Int Reason4/1 -> FIFO read 2/2
  Xmt 2/1 -> FIFO read 2/1
  FIFO read 2/1 -> Write HW FIFO2/1
  FIFO read 2/2 -> Write HW FIFO2/2
  FIFO read 1/1 -> Write HW FIFO1/1
  FIFO read 1/2 -> Write HW FIFO1/2
  Constant1/1 -> FIFO read 1/3
  Constant2/1 -> FIFO read 2/3
  Logical Operator/1 -> While Iterator/1
  Relational Operator/1 -> Logical Operator/1
  Bitwise Logical Operator/1 -> Relational Operator/2
  Constant9/1 -> Relational Operator/1

== system xpclib/RS232/Quatech/ESC-100/ESC-100/RS232 ISR ==
  Xmt 1 : Inport  LatchInput=off
  Xmt 2 : Inport  Port=2  LatchInput=off
  Xmt 3 : Inport  Port=3  LatchInput=off
  Xmt 4 : Inport  Port=4  LatchInput=off
  Xmt 5 : Inport  Port=5  LatchInput=off
  Xmt 6 : Inport  Port=6  LatchInput=off
  Xmt 7 : Inport  Port=7  LatchInput=off
  Xmt 8 : Inport  Port=8  LatchInput=off
  function : TriggerPort  TriggerType=function-call
  While Iterator Subsystem : Subsystem  TreatAsAtomicUnit=on  PropExecContextAcrossSSBoundary=on
  Recv 1 : Outport
  Recv 2 : Outport  Port=2
  Recv 3 : Outport  Port=3
  Recv 4 : Outport  Port=4
  Recv 5 : Outport  Port=5
  Recv 6 : Outport  Port=6
  Recv 7 : Outport  Port=7
  Recv 8 : Outport  Port=8
  wires:
  Xmt 1/1 -> While Iterator Subsystem/1(Xmt 1)
  Xmt 2/1 -> While Iterator Subsystem/2(Xmt 2)
  Xmt 3/1 -> While Iterator Subsystem/3(Xmt 3)
  Xmt 4/1 -> While Iterator Subsystem/4(Xmt 4)
  Xmt 5/1 -> While Iterator Subsystem/5(Xmt 5)
  Xmt 6/1 -> While Iterator Subsystem/6(Xmt 6)
  Xmt 7/1 -> While Iterator Subsystem/7(Xmt 7)
  Xmt 8/1 -> While Iterator Subsystem/8(Xmt 8)
  While Iterator Subsystem/1(Recv 1) -> Recv 1/1
  While Iterator Subsystem/2(Recv 2) -> Recv 2/1
  While Iterator Subsystem/3(Recv 3) -> Recv 3/1
  While Iterator Subsystem/4(Recv 4) -> Recv 4/1
  While Iterator Subsystem/5(Recv 5) -> Recv 5/1
  While Iterator Subsystem/6(Recv 6) -> Recv 6/1
  While Iterator Subsystem/7(Recv 7) -> Recv 7/1
  While Iterator Subsystem/8(Recv 8) -> Recv 8/1

== system xpclib/RS232/Quatech/QSC-100/QSC-100/RS232 ISR ==
  Xmt 1 : Inport  LatchInput=off
  Xmt 2 : Inport  Port=2  LatchInput=off
  Xmt 3 : Inport  Port=3  LatchInput=off
  Xmt 4 : Inport  Port=4  LatchInput=off
  function : TriggerPort  TriggerType=function-call
  While Iterator Subsystem : Subsystem  TreatAsAtomicUnit=on  PropExecContextAcrossSSBoundary=on
  Recv 1 : Outport
  Recv 2 : Outport  Port=2
  Recv 3 : Outport  Port=3
  Recv 4 : Outport  Port=4
  wires:
  Xmt 1/1 -> While Iterator Subsystem/1(Xmt 1)
  Xmt 2/1 -> While Iterator Subsystem/2(Xmt 2)
  Xmt 3/1 -> While Iterator Subsystem/3(Xmt 3)
  Xmt 4/1 -> While Iterator Subsystem/4(Xmt 4)
  While Iterator Subsystem/1(Recv 1) -> Recv 1/1
  While Iterator Subsystem/2(Recv 2) -> Recv 2/1
  While Iterator Subsystem/3(Recv 3) -> Recv 3/1
  While Iterator Subsystem/4(Recv 4) -> Recv 4/1

== system xpclib/RS232/Quatech/QSC-200/300/QSC-200/300 /RS232 ISR ==
  Xmt 1 : Inport  LatchInput=off
  Xmt 2 : Inport  Port=2  LatchInput=off
  Xmt 3 : Inport  Port=3  LatchInput=off
  Xmt 4 : Inport  Port=4  LatchInput=off
  function : TriggerPort  TriggerType=function-call
  While Iterator Subsystem : Subsystem  TreatAsAtomicUnit=on  PropExecContextAcrossSSBoundary=on
  Recv 1 : Outport
  Recv 2 : Outport  Port=2
  Recv 3 : Outport  Port=3
  Recv 4 : Outport  Port=4
  wires:
  Xmt 1/1 -> While Iterator Subsystem/1(Xmt 1)
  Xmt 2/1 -> While Iterator Subsystem/2(Xmt 2)
  Xmt 3/1 -> While Iterator Subsystem/3(Xmt 3)
  Xmt 4/1 -> While Iterator Subsystem/4(Xmt 4)
  While Iterator Subsystem/1(Recv 1) -> Recv 1/1
  While Iterator Subsystem/2(Recv 2) -> Recv 2/1
  While Iterator Subsystem/3(Recv 3) -> Recv 3/1
  While Iterator Subsystem/4(Recv 4) -> Recv 4/1

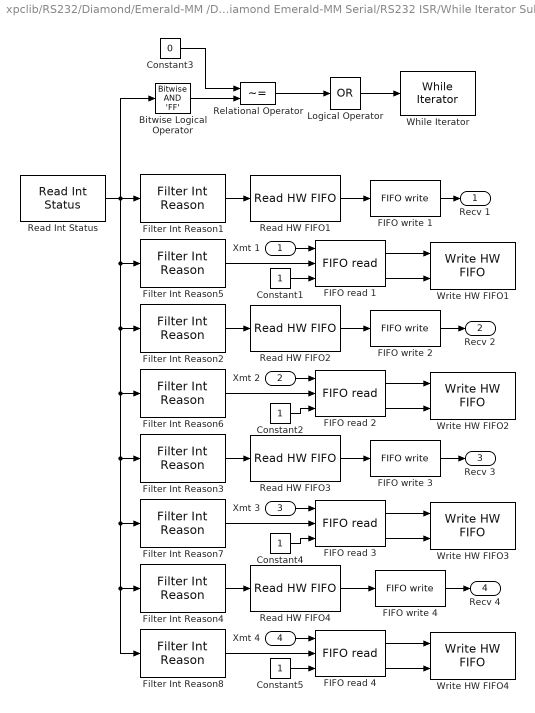
== system xpclib/RS232/Diamond/Emerald-MM /Diamond Emerald-MM Serial/RS232 ISR/While Iterator Subsystem ==
  Xmt 1 : Inport  LatchInput=off
  Xmt 2 : Inport  Port=2  LatchInput=off
  Xmt 3 : Inport  Port=3  LatchInput=off
  Xmt 4 : Inport  Port=4  LatchInput=off
  Bitwise Logical Operator : simulink/Logic and Bit Operations/Bitwise Operator  logicop=AND  UseBitMask=on  BitMask='FF'  BitMaskRealWorld=Stored Integer
  Constant{1..2,4..5} (4 alike) : Constant  OutDataTypeMode=uint32
  Constant3 : Constant  Value=0  OutDataTypeMode=uint32
  FIFO read {1..4} (4 alike) : xpclib/RS232/FIFO read   maxsize=60  minsize=1  usedelimiter=off  delimiter=13  outputtype=count+32 bit uint  enable=on  enableout=on  sampletime=-1
  FIFO write 1 : xpclib/RS232/FIFO write   size=1024  inputtype=count+32 bit uint  present=off  sampletime=-1  id=RCV channel 1, IRQ 7
  FIFO write 2 : xpclib/RS232/FIFO write   size=1024  inputtype=count+32 bit uint  present=off  sampletime=-1  id=RCV channel 2, IRQ 7
  FIFO write 3 : xpclib/RS232/FIFO write   size=1024  inputtype=count+32 bit uint  present=off  sampletime=-1  id=RCV channel 3, IRQ 7
  FIFO write 4 : xpclib/RS232/FIFO write   size=1024  inputtype=count+32 bit uint  present=off  sampletime=-1  id=RCV channel 4, IRQ 7
  Filter Int Reason1 : xpclib/RS232/Diamond/Emerald-MM /Diamond Emerald-MM/Filter Int Reason  port=1  value=Receive data
  Filter Int Reason2 : xpclib/RS232/Diamond/Emerald-MM /Diamond Emerald-MM/Filter Int Reason  port=2  value=Receive data
  Filter Int Reason3 : xpclib/RS232/Diamond/Emerald-MM /Diamond Emerald-MM/Filter Int Reason  port=3  value=Receive data
  Filter Int Reason4 : xpclib/RS232/Diamond/Emerald-MM /Diamond Emerald-MM/Filter Int Reason  port=4  value=Receive data
  Filter Int Reason5 : xpclib/RS232/Diamond/Emerald-MM /Diamond Emerald-MM/Filter Int Reason  port=1  value=Transmitter empty
  Filter Int Reason6 : xpclib/RS232/Diamond/Emerald-MM /Diamond Emerald-MM/Filter Int Reason  port=2  value=Transmitter empty
  Filter Int Reason7 : xpclib/RS232/Diamond/Emerald-MM /Diamond Emerald-MM/Filter Int Reason  port=3  value=Transmitter empty
  Filter Int Reason8 : xpclib/RS232/Diamond/Emerald-MM /Diamond Emerald-MM/Filter Int Reason  port=4  value=Transmitter empty
  Logical Operator : Logic  Operator=OR  Inputs=1  AllPortsSameDT=off
  Read HW FIFO1 : xpclib/RS232/Diamond/Emerald-MM /Diamond Emerald-MM/Read HW FIFO  flush=on  addr=baddr1
  Read HW FIFO2 : xpclib/RS232/Diamond/Emerald-MM /Diamond Emerald-MM/Read HW FIFO  flush=on  addr=baddr2
  Read HW FIFO3 : xpclib/RS232/Diamond/Emerald-MM /Diamond Emerald-MM/Read HW FIFO  flush=on  addr=baddr3
  Read HW FIFO4 : xpclib/RS232/Diamond/Emerald-MM /Diamond Emerald-MM/Read HW FIFO  flush=on  addr=baddr4
  Read Int Status : xpclib/RS232/Diamond/Emerald-MM /Diamond Emerald-MM/Read Int Status  addr1=baddr1  addr2=baddr2  addr3=baddr3  addr4=baddr4  intstat=istat
  Relational Operator : RelationalOperator  Operator=~=
  While Iterator : WhileIterator  MaxIters=66  WhileBlockType=do-while
  Write HW FIFO1 : xpclib/RS232/Diamond/Emerald-MM /Diamond Emerald-MM/Write HW FIFO  addr=baddr1
  Write HW FIFO2 : xpclib/RS232/Diamond/Emerald-MM /Diamond Emerald-MM/Write HW FIFO  addr=baddr2
  Write HW FIFO3 : xpclib/RS232/Diamond/Emerald-MM /Diamond Emerald-MM/Write HW FIFO  addr=baddr3
  Write HW FIFO4 : xpclib/RS232/Diamond/Emerald-MM /Diamond Emerald-MM/Write HW FIFO  addr=baddr4
  Recv 1 : Outport
  Recv 2 : Outport  Port=2
  Recv 3 : Outport  Port=3
  Recv 4 : Outport  Port=4
  wires:
  FIFO read 2/2 -> Write HW FIFO2/2
  FIFO read 2/1 -> Write HW FIFO2/1
  FIFO read 3/2 -> Write HW FIFO3/2
  FIFO read 3/1 -> Write HW FIFO3/1
  FIFO read 4/2 -> Write HW FIFO4/2
  FIFO read 4/1 -> Write HW FIFO4/1
  Filter Int Reason4/1 -> Read HW FIFO4/1
  Read HW FIFO3/1 -> FIFO write 3/1
  Filter Int Reason3/1 -> Read HW FIFO3/1
  Filter Int Reason2/1 -> Read HW FIFO2/1
  Read HW FIFO4/1 -> FIFO write 4/1
  Filter Int Reason1/1 -> Read HW FIFO1/1
  Filter Int Reason6/1 -> FIFO read 2/2
  Filter Int Reason7/1 -> FIFO read 3/2
  Filter Int Reason8/1 -> FIFO read 4/2
  Xmt 3/1 -> FIFO read 3/1
  Xmt 4/1 -> FIFO read 4/1
  Constant4/1 -> FIFO read 3/3
  Constant5/1 -> FIFO read 4/3
  FIFO write 3/1 -> Recv 3/1
  FIFO write 4/1 -> Recv 4/1
  Logical Operator/1 -> While Iterator/1
  Relational Operator/1 -> Logical Operator/1
  Read Int Status/1 -> Filter Int Reason4/1, Filter Int Reason8/1, Filter Int Reason7/1, Filter Int Reason3/1, Filter Int Reason6/1, Filter Int Reason2/1, Filter Int Reason5/1, Bitwise Logical Operator/1, Filter Int Reason1/1
  FIFO write 1/1 -> Recv 1/1
  Read HW FIFO1/1 -> FIFO write 1/1
  Filter Int Reason5/1 -> FIFO read 1/2
  Xmt 1/1 -> FIFO read 1/1
  FIFO write 2/1 -> Recv 2/1
  Read HW FIFO2/1 -> FIFO write 2/1
  Xmt 2/1 -> FIFO read 2/1
  FIFO read 1/1 -> Write HW FIFO1/1
  FIFO read 1/2 -> Write HW FIFO1/2
  Constant1/1 -> FIFO read 1/3
  Constant2/1 -> FIFO read 2/3
  Bitwise Logical Operator/1 -> Relational Operator/2
  Constant3/1 -> Relational Operator/1
